simulink model "AOCS_FDIR"  (R2020b)
settings: Solver=ode45  StartTime=0.0  StopTime=200  FixedStep=1e-4  MaxStep=0.25  RelTol=1e-8  AbsTol=1e-8
values from neighbouring files (symbols this model uses):
  Gyros = zeros(3,6)    [Generate_Data.m]
  ReWhe = zeros(3,4)    [Generate_Data.m]
  Thrus = ones(1,8)    [Generate_Data.m]
undefined symbols (not defined in the file or in its folder): A, A_FEEP, A_FEEP_real, A_mag, CG_real, d_face, Dipole_SC, e0_0, e1_0, e2_0, e3_0, e_max_att, e_max_orb, Env_Drag, Env_J2, Env_Moon, Env_Sun, Env_TGG, Env_TMag, FEEP, g, GNSS, gyr, h_ref, h_RW, h_rw_0, I, I_real, IAU, initial_date_JD, J2, K_det, k_quat, km, m, mag, mu, mu_Moon, mu_Sun, n, n_orbits, q_0, Re, RW1, RW2, RW3, RW4, rx0, ry0, rz0, s, sigma1, sigma2, star, T_friction, th_2_gyr, th_FR_gyr, th_RW, th_SD_gyr_null, th_thruster ... (+10)
libraries: dspstat3 x16, aerolibutil x8, sharedutil x6, sharedtransform x5, vrlib x3, aerolibtransform2 x3, aerolibcelestial x2, aerolibobsolete x1, dspinverses x1
(part 4 of 4)

== matlab function AOCS_FDIR/Visualization/3D Orbit/3D Orbit Plot ==
  settings: updateMethod=DISCRETE
  data: x input; v input; DCM input; time input
function fcn(x,v,DCM,time)

persistent initialize;
persistent pc1;
persistent pc2;
persistent pc3;
persistent pc4;
persistent pc5;
persistent pc6;
persistent pc7;
persistent pc8;
persistent pc9;
persistent pc10;
persistent pc11;
persistent pc12;
persistent pc13;
persistent pc14;
persistent th;
persistent th1;
persistent th2;
persistent th3;
persistent time0;
persistent globe;
persistent orbit;
% persistent i_LVLH;
% persistent j_LVLH;
% persistent k_LVLH;

coder.extrinsic('patch');
coder.extrinsic('delete')
coder.extrinsic('earth_example')
coder.extrinsic('mArrow3')
coder.extrinsic('cylinder2P')
coder.extrinsic('ellipsoid')
coder.extrinsic('imread')
coder.extrinsic('rotate')
coder.extrinsic('animatedline')
coder.extrinsic('addpoints')

if isempty(initialize)
    figure(1)
    axes('Units', 'normalized', 'Position', [0 0 1 1])
    hold on
    
    % Customize the window
    set(gcf,'Menubar','none','Name','3D Orbit', ...
        'NumberTitle','off','Position',[0,0,825,840], ...
        'Color',[0 0 0]);
    
    % Plot the Earth in the correct position
    npanels = 180;
    erad    = 6378137;
    prad    = 6356752.31424518;
    [x, y, z] = ellipsoid(0, 0, 0, erad, erad, prad, npanels);
    
    image_file = 'ModifiedBlueMarble.jpg';
    
    globe=surf(x, y, -1*z, 'FaceColor', 'none', 'EdgeColor', 0.5*[1 1 1]);
    
    cdata = imread(image_file);
    set(globe, 'FaceColor', 'texturemap', 'CData', cdata, 'FaceAlpha', 1, 'EdgeColor', 'none');
    material(globe,'dull')
    
    set(gcf,'Color','k');
    
    % Plot ECI frame
    b = 9000000;
    mArrow3([0 0 0],b*[1 0 0]','color','yellow','stemWidth',1e5);
    mArrow3([0 0 0],b*[0 1 0]','color','yellow','stemWidth',1e5);
    mArrow3([0 0 0],b*[0 0 1]','color','yellow','stemWidth',1e5);
    text(b,0,0.15*b,'x','Color','y')
    text(0,b,0.15*b,'y','Color','y')
    text(0,0.1*b,b,'z','Color','y')
    
    % Customize the view 
    view(135,20);
    light('Position',[2,0.5,0.5]);
    lighting gouraud; 
    axis off;
    axis equal;
    axis([-10000000 10000000 -10000000 10000000 -10000000 10000000])
 
    initialize = 1;
    pc1        = patch(1e6*[0 0 1 1],1e6*[0 1 1 0],1e6*[1 1 1 1],'b');
    pc2        = patch(1e6*[0 0 1 1],1e6*[0 1 1 0],1e6*[1 1 1 1],'b');
    pc3        = patch(1e6*[0 0 1 1],1e6*[0 1 1 0],1e6*[1 1 1 1],'b');
    pc4        = patch(1e6*[0 0 1 1],1e6*[0 1 1 0],1e6*[1 1 1 1],'b');
    pc5        = patch(1e6*[0 0 1 1],1e6*[0 1 1 0],1e6*[1 1 1 1],'b');
    pc6        = patch(1e6*[0 0 1 1],1e6*[0 1 1 0],1e6*[1 1 1 1],'b');
    pc7        = patch(1e6*[0 0 1 1],1e6*[0 1 1 0],1e6*[1 1 1 1],'b');
    pc8        = patch(1e6*[0 0 1 1],1e6*[0 1 1 0],1e6*[1 1 1 1],'b');
    pc9        = patch(1e6*[0 0 1 1],1e6*[0 1 1 0],1e6*[1 1 1 1],'b');
    pc10       = patch(1e6*[0 0 1 1],1e6*[0 1 1 0],1e6*[1 1 1 1],'b');
    pc11       = patch(1e6*[0 0 1 1],1e6*[0 1 1 0],1e6*[1 1 1 1],'b');
    pc12       = patch(1e6*[0 0 1 1],1e6*[0 1 1 0],1e6*[1 1 1 1],'b');
    pc13       = patch(1e6*[0 0 1 1],1e6*[0 1 1 0],1e6*[1 1 1 1],'b');
    pc14       = patch(1e6*[0 0 1 1],1e6*[0 1 1 0],1e6*[1 1 1 1],'b');
    th         = patch(1e6*[0 0 1 1],1e6*[0 1 1 0],1e6*[1 1 1 1],'b');
    th1        = patch(1e6*[0 0 1 1],1e6*[0 1 1 0],1e6*[1 1 1 1],'b');
    th2        = patch(1e6*[0 0 1 1],1e6*[0 1 1 0],1e6*[1 1 1 1],'b');
    th3        = patch(1e6*[0 0 1 1],1e6*[0 1 1 0],1e6*[1 1 1 1],'b');
    
    rotate(globe,[0 0 -1],22, [0 0 0]);
    orbit = animatedline('Color','r');
    time0 = 0;
    
else
    figure(1)
    rotate(globe,[0 0 1],(time-time0)*360/86400, [0 0 0]);
    
    ll = 5e5;
    %czoom = 13;
    
    delete(pc1)
    delete(pc2)
    delete(pc3)
    delete(pc4)
    delete(pc5)
    delete(pc6)
    delete(pc7)
    delete(pc8)
    delete(pc9)
    delete(pc10)
    delete(pc11)
    delete(pc12)
    delete(pc13)
    delete(pc14)
    delete(th)
    delete(th1)
    delete(th2)
    delete(th3)
    
    ii = x/sqrt(x(1)^2+x(2)^2+x(3)^2);
    jj = v/sqrt(v(1)^2+v(2)^2+v(3)^2);
    
    % Plot the orbit
    addpoints(orbit,x(1),x(2),x(3));
    
    %plot3(x(1),x(2),x(3),'ro','MarkerSize',2)
    %plot3(x_des(1),x_des(2),x_des(3),'bo','MarkerSize',1)
    
    % Satellite
    
    vpc1  = [ll*[0.5 0.5 0.5 0.5];2*ll*[-0.5 -0.5 0.5 0.5]; ll*[-0.5 0.5 0.5 -0.5]];
    vpc2  = [ll*[-0.5 -0.5 -0.5 -0.5];2*ll*[-0.5 -0.5 0.5 0.5];ll*[-0.5 0.5 0.5 -0.5]];
    vI1   = 0.6*DCM'*vpc1;
    vI2   = 0.6*DCM'*vpc2;
    
    pc1 = patch(x(1)+vI1(1,:),x(2)+vI1(2,:),x(3)+vI1(3,:),'blue');
    pc2 = patch(x(1)+vI2(1,:),x(2)+vI2(2,:),x(3)+vI2(3,:),'blue');
    %
    
    vpc1  = [ll*[0.5 0.5 -0.5 -0.5];2*ll*[-0.5 0.5  0.5 -0.5];ll*[-0.5 -0.5 -0.5 -0.5]];
    vpc2  = [ll*[0.5 0.5 -0.5 -0.5];2*ll*[-0.5 0.5  0.5 -0.5];ll*[ 0.5  0.5  0.5  0.5]];
    vI1   = 0.6*DCM'*vpc1;
    vI2   = 0.6*DCM'*vpc2;
    
    pc3 = patch(x(1)+vI1(1,:),x(2)+vI1(2,:),x(3)+vI1(3,:),'blue');
    pc4 = patch(x(1)+vI2(1,:),x(2)+vI2(2,:),x(3)+vI2(3,:),'blue');
    %
    vpc1  = [ll*[0.5 0.5 -0.5 -0.5];2*ll*[0.5 0.5  0.5 0.5];ll*[ 0.5 -0.5 -0.5 0.5]];
    vpc2  = [ll*[0.5 0.5 -0.5 -0.5];2*ll*[-0.5 -0.5  -0.5 -0.5];ll*[ 0.5  -0.5  -0.5  0.5]];
    vI1   = 0.6*DCM'*vpc1;
    vI2   = 0.6*DCM'*vpc2;
    
    pc5 = patch(x(1)+vI1(1,:),x(2)+vI1(2,:),x(3)+vI1(3,:),'blue');
    pc6 = patch(x(1)+vI2(1,:),x(2)+vI2(2,:),x(3)+vI2(3,:),'blue');
    
    % Solar Panel 
%     vB1  = [ll*[0 0 0 0];ll*[1 3 3 1]; ll*[ -0.5 -0.5 +0.5 0.5]];
%     vB2  = [ll*[0 0 0 0];ll*[-1 -3 -3 -1];ll*[ -0.5 -0.5  +0.5 0.5]];
%     vI1   = 0.6*DCM'*vB1;
%     vI2   = 0.6*DCM'*vB2;
    
    %pc7 = patch(x(1)+vI1(1,:),x(2)+vI1(2,:),x(3)+vI1(3,:),'white');
    %pc8 = patch(x(1)+vI2(1,:),x(2)+vI2(2,:),x(3)+vI2(3,:),'white');
    
%     % THRUSTER
%     r   = ll/4;
%     r1  = (ll*[-0.5, -0.5, -0.5] + ll*[-0.5, 0.5, 0.5])/2;
%     vr1 = x + DCM'*r1';
%     vr2 = vr1 - ll/3*DCM(1,:)';
%     
%     [X, Y, Z] = cylinder2P(r, 20,vr1',vr2');
%         th=surf(X,Y,Z,'facecolor','white');
%     [X, Y, Z] = cylinder2P(ll/5, 40,vr1',(vr2- ll/8*DCM(1,:)')');
%         th1=surf(X,Y,Z,'facecolor','red');
%     [X, Y, Z] = cylinder2P(ll/6, 40,vr1',(vr2-ll/5*DCM(1,:)')');
%         th2=surf(X,Y,Z,'facecolor','red');
%     [X, Y, Z] = cylinder2P(ll/7, 40,vr1',(vr2- ll/3*DCM(1,:)')');
%         th3=surf(X,Y,Z,'facecolor','red');
    
    % LVLH
    k_LVLH = -x/norm(x);
    j_LVLH = -cross(x,v)/norm(cross(x,v));
    i_LVLH = cross(j_LVLH,k_LVLH);
    pc9  = mArrow3(x,x + ll*1.8*i_LVLH,'color','yellow','stemWidth',ll/20);
    pc10 = mArrow3(x,x + ll*1.8*j_LVLH,'color','yellow','stemWidth',ll/20);
    pc11 = mArrow3(x,x + ll*1.8*k_LVLH,'color','yellow','stemWidth',ll/20);
    
    % BODY FRAME
    pc12 = mArrow3(x,x + ll*1.8*DCM(1,:)','color','cyan','stemWidth',ll/20);
    pc13 = mArrow3(x,x + ll*1.8*DCM(2,:)','color','red','stemWidth',ll/20);
    pc14 = mArrow3(x,x + ll*1.8*DCM(3,:)','color','green','stemWidth',ll/20);
    
    %xlim([-20e7 20e7])
    %ylim([-20e7 20e7])
    %zlim([-20e7 20e7])
    
    material(pc1,'dull')
    material(pc2,'dull')
    material(pc3,'dull')
    material(pc4,'dull')
    material(pc5,'dull')
    material(pc6,'dull')
    material(pc7,'metal')
    material(pc8,'metal')
    material(th,'metal')
    
    %campos([x(1)+czoom*ll*ii(1),x(2)+czoom*ll*ii(2),x(3)+czoom*ll*ii(3)]) % vista segun r
    %campos([x(1),x(2),x(3)+czoom*ll]) % vista de arriba
    % segun vector velocidad
    %campos([x(1)+czoom*ll*jj(1),x(2)+czoom*ll*jj(2),x(3)+czoom*ll*jj(3)])
    
    
    %camtarget([x(1),x(2),x(3)])
    %camtarget([0,0,0])
   
    %camva(80)
    %earth_example
    
    time0 = time;
    
    drawnow
end

== matlab function AOCS_FDIR/Visualization/Groundtrack/Groundtrack ==
  settings: updateMethod=DISCRETE
  data: lat input; lon input
function fcn(lat, lon)

persistent initialize;
persistent groundtrack;
persistent lon0;
persistent sat1;
persistent sat2;
persistent sat3;
persistent sat4;

coder.extrinsic('animatedline')
coder.extrinsic('addpoints')
coder.extrinsic('imread')
coder.extrinsic('imagesc')
coder.extrinsic('delete')
coder.extrinsic('patch')
coder.extrinsic('line')

if isempty(initialize)
     figure(2)
    % Customize the window
    set(gcf,'Menubar','none','Name','Groundtrack', ...
        'NumberTitle','off','Position',[825,42,710,355], ...
        'Color',[1 1 1]);

    % Plot the worldmap
    img = imread('ModifiedBlueMarble.jpg');
    
    min_x = -180;
    max_x = 180;
    min_y = -90;
    max_y = 90;
    
    imagesc([min_x max_x], [min_y max_y], flipud(img));
    lon0 = lon;
    
    % Customize the view
    set(gca,'Ydir','default','GridColor','k','GridAlpha',0.4,...
        'XTick',-180:30:180,'YTick',-90:30:90)
    axis([min_x,max_x,min_y, max_y])
    grid on;
    
    sat1        = patch([1 0 -1 0]*2.75+lon,[0 1 0 -1]*2.75+lat,'k');
    sat2        = line([-0.75 0.75]*2.75+lon,[0.75,-0.75]*2.75+lat,'Color','k');
    sat3        = patch([-1 -0.5 -2 -2.5]*2.75+lon, [0.5 1 2.5 2]*2.75+lat,'white');
    sat4        = patch([-1 -0.5 -2 -2.5]*-2.75+lon, [0.5 1 2.5 2]*-2.75+lat,'white');
    initialize  = 1;
    groundtrack = animatedline('Color','r');
    
else     
    figure(2)
    delete(sat1)
    delete(sat2)
    delete(sat3)
    delete(sat4)
    
    if sind(lon0)*sind(lon)<=0
        groundtrack = animatedline('Color','r');
        addpoints(groundtrack,lon,lat);
    else
        addpoints(groundtrack,lon,lat);
    end
    
    sat1 = patch([1 0 -1 0]*2.5+lon,[0 1 0 -1]*2.5+lat,'k');
    sat2 = line([-0.75 0.75]*2.5+lon,[0.75,-0.75]*2.5+lat,'Color','k');
    sat3 = patch([-1 -0.5 -1.5 -2]*2.5+lon, [0.5 1 2 1.5]*2.5+lat,'white');
    sat4 = patch([-1 -0.5 -1.5 -2]*-2.5+lon, [0.5 1 2 1.5]*-2.5+lat,'white');
      
    lon0 = lon;
    drawnow
end
